simulink model "motor_model"  (Simulink 9.1)
settings: Solver=VariableStepAuto  StartTime=0.0  StopTime=10.0  RelTol=1e-3
settings Model: Creator=PSere  LastModifiedBy=PSere
settings DataIOCC: SaveFormat=Dataset
settings OptimizationCC: LifeSpan=auto
settings DebuggingCC: UnderspecifiedInitializationDetection=Simplified  MergeDetectMultiDrivingBlocksExec=error  SFUnexpectedBacktrackingDiag=error  SFNoUnconditionalDefaultTransitionDiag=error  SFExecutionAtInitializationDiag=warning
settings HardwareCC: ProdBitPerPointer=64  ProdBitPerSizeT=64  ProdBitPerPtrDiffT=64  ProdLargestAtomicFloat=Float  ProdIntDivRoundTo=Zero  ProdEndianess=LittleEndian  ProdWordSize=64  ProdHWDeviceType=Intel->x86-64 (Windows64)
settings ModelReferenceCC: PropagateSignalLabelsOutOfModel=on
settings CodeAppCC: StateflowObjectComments=off
settings GRTTargetCC: TargetLangStandard=C99 (ISO)  CombineOutputUpdateFcns=on  GRTInterface=off
settings ConfigComp: CovMetricSettings=dwe  CovHtmlReporting=off  CovSaveCumulativeToWorkspaceVar=off  CovSaveSingleToWorkspaceVar=off  CovExternalEMLEnable=on

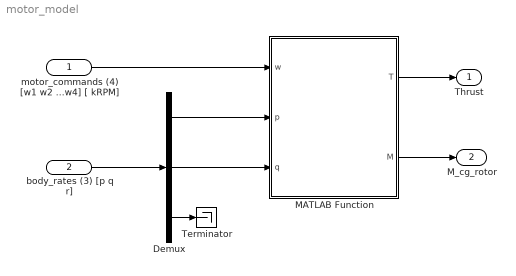
== system motor_model ==
  motor_commands (4) [w1 w2 w3 w4] [ kRPM] : Inport
  body_rates (3) [p q r] : Inport  Port=2
  Demux : Demux  Outputs=3
  MATLAB Function : MATLAB Function  TreatAsAtomicUnit=on
  Terminator : Terminator
  Thrust : Outport
  M_cg_rotor : Outport  Port=2
  wires:
  motor_commands (4) [w1 w2 w3 w4] [ kRPM]/1 -> MATLAB Function/1(w)
  MATLAB Function/1(T) -> Thrust/1
  MATLAB Function/2(M) -> M_cg_rotor/1
  body_rates (3) [p q r]/1 -> Demux/1
  Demux/2 -> MATLAB Function/3(q)
  Demux/1 -> MATLAB Function/2(p)
  Demux/3 -> Terminator/1

== matlab function MATLAB Function ==
  data: w input double; T output double; M output double; p input double; q input double
function [T, M] = motor_model(w, p, q)
%% Deltaquad Parameters:
      
Irzz    = 0.05;                            % rotor inertia
dx      = 0.35;                            % position of rotors x
dy      = 0.35;                            % position of rotors y
k1      = 12.2625;                         % N / kRPM^2
k2      = 4.2;                             % Nm / kRPM^2

%% Thrust and Moments:
% 1) Total Thrust body axis
T = -k1 * sum(w.^2);

% 2) Mc: Conrol moments:
Mc = [-dy*k1, dy*k1,  dy*k1, -dy*k1;
       dx*k1, dx*k1, -dx*k1, -dx*k1;
       k2,    -k2,    k2,      -k2]*w.^2;
   
% 3) Mr: Gyroscopic effect:
Mr = [ Irzz*q, -Irzz*q,  Irzz*q, -Irzz*q;
      -Irzz*p,  Irzz*p, -Irzz*p,  Irzz*p;
            0,       0,       0,       0]*w;

M = Mc - Mr;
